simulink model "motorsubsystem"  (R2024b)
settings: Solver=VariableStepAuto  StartTime=0.0  StopTime=10.0  RelTol=1e-3
values from neighbouring files (symbols this model uses):
  b = 0.00068    [matlab.mat]
  J = 0.01    [matlab.mat]
  ke = 0.229    [matlab.mat]
  kt = 0.11864    [matlab.mat]
  L = 0.001    [matlab.mat]
  R = 2.4    [matlab.mat]
settings Model: Creator=omari  LastModifiedBy=omari

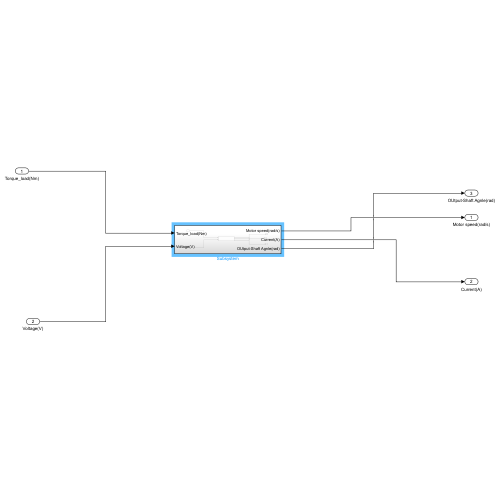
[thumbnail: Simulink's stored preview of the top-level diagram]
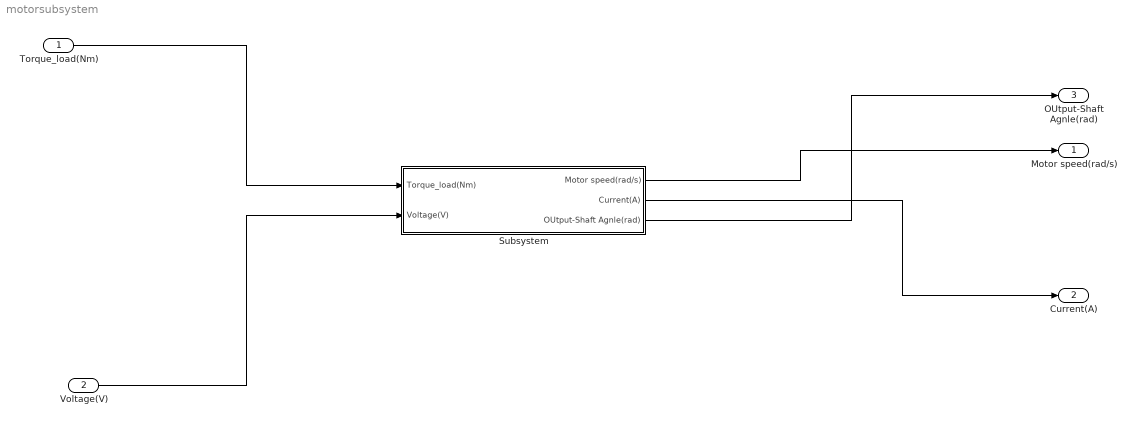
== system motorsubsystem ==
  Torque_load(Nm) : Inport
  Voltage(V) : Inport  Port=2
  Subsystem : Subsystem
  Motor speed(rad/s) : Outport
  Current(A) : Outport  Port=2
  OUtput-Shaft Agnle(rad) : Outport  Port=3
  wires:
  Torque_load(Nm)/1 -> Subsystem/1(Torque_load(Nm))
  Voltage(V)/1 -> Subsystem/2(Voltage(V))
  Subsystem/1(Motor speed(rad/s)) -> Motor speed(rad/s)/1
  Subsystem/2(Current(A)) -> Current(A)/1
  Subsystem/3(OUtput-Shaft Agnle(rad)) -> OUtput-Shaft Agnle(rad)/1

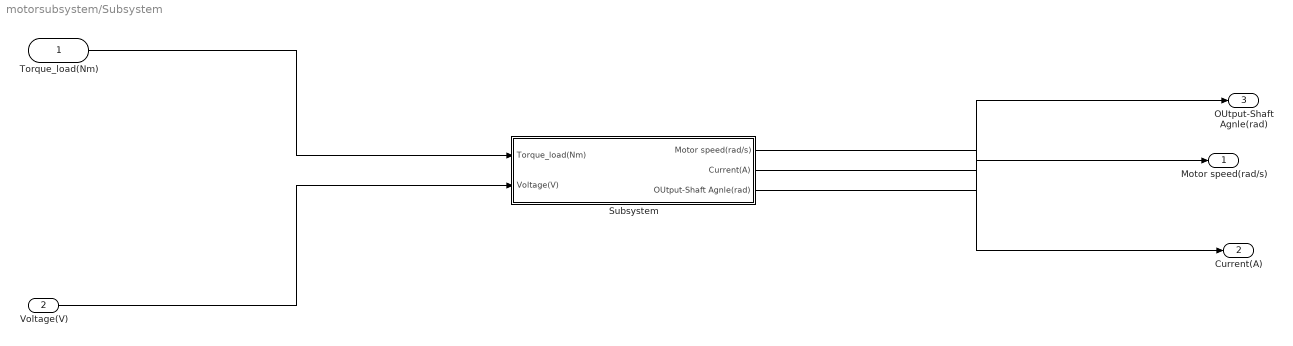
== system motorsubsystem/Subsystem ==
  Torque_load(Nm) : Inport
  Voltage(V) : Inport  Port=2
  Subsystem : Subsystem
  Motor speed(rad/s) : Outport
  Current(A) : Outport  Port=2
  OUtput-Shaft Agnle(rad) : Outport  Port=3
  wires:
  Torque_load(Nm)/1 -> Subsystem/1(Torque_load(Nm))
  Voltage(V)/1 -> Subsystem/2(Voltage(V))
  Subsystem/1(Motor speed(rad/s)) -> Motor speed(rad/s)/1
  Subsystem/2(Current(A)) -> Current(A)/1
  Subsystem/3(OUtput-Shaft Agnle(rad)) -> OUtput-Shaft Agnle(rad)/1

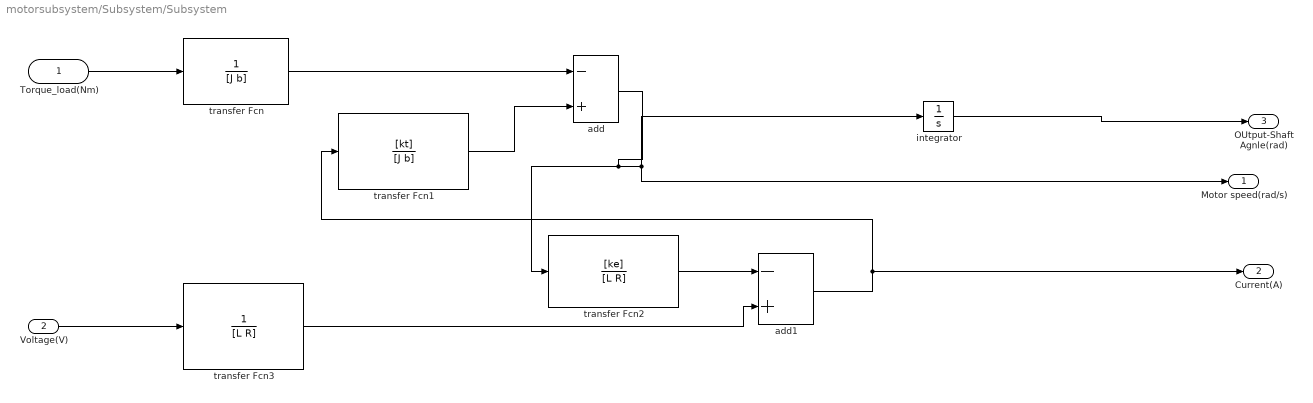
== system motorsubsystem/Subsystem/Subsystem ==
  Torque_load(Nm) : Inport
  Voltage(V) : Inport  Port=2
  add : Sum  Inputs=-+
  add1 : Sum  Inputs=-+
  integrator : Integrator
  transfer Fcn : TransferFcn  Denominator=[J b]
  transfer Fcn1 : TransferFcn  Numerator=[kt]  Denominator=[J b]
  transfer Fcn2 : TransferFcn  Numerator=[ke]  Denominator=[L R]
  transfer Fcn3 : TransferFcn  Denominator=[L R]
  Motor speed(rad/s) : Outport
  Current(A) : Outport  Port=2
  OUtput-Shaft Agnle(rad) : Outport  Port=3
  wires:
  add/1 -> transfer Fcn2/1, Motor speed(rad/s)/1, integrator/1
  add1/1 -> Current(A)/1, transfer Fcn1/1
  Torque_load(Nm)/1 -> transfer Fcn/1
  transfer Fcn3/1 -> add1/2
  transfer Fcn2/1 -> add1/1
  Voltage(V)/1 -> transfer Fcn3/1
  transfer Fcn/1 -> add/1
  transfer Fcn1/1 -> add/2
  integrator/1 -> OUtput-Shaft Agnle(rad)/1
